simulink model "SwitchingFrequencyControlComponent"  (R2026a)
settings: Solver=FixedStepDiscrete
settings Model: DataDictionary=TractionEmotorSoftwareArchInterfaceData.sldd  Creator=dakaihu  LastModifiedBy=dakaihu

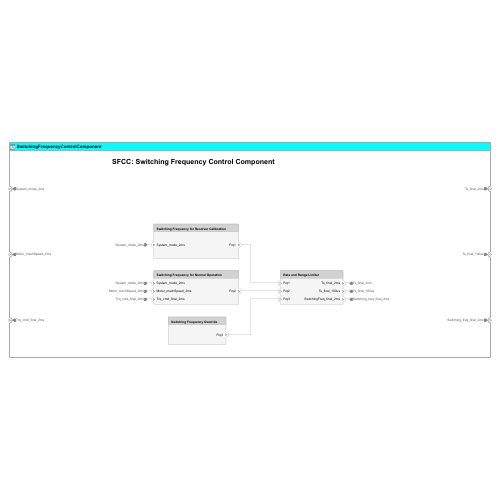
[thumbnail: Simulink's stored preview of the top-level diagram]
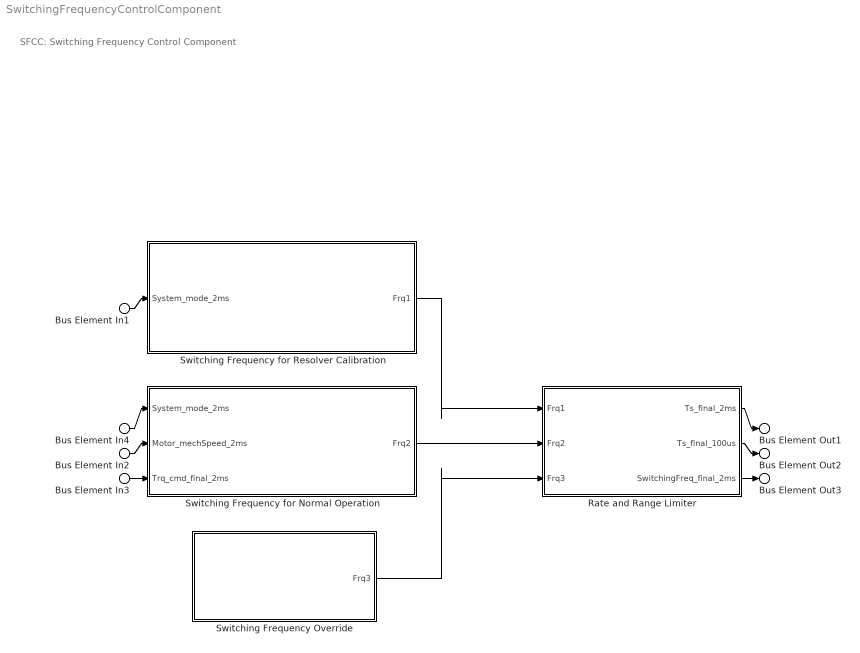
== system SwitchingFrequencyControlComponent ==
  note: SFCC: Switching Frequency Control Component
  Bus Element In1 : Inport  PortName=System_mode_2ms
  Bus Element In4 : Inport  PortName=System_mode_2ms
  Bus Element In2 : Inport  Port=2  PortName=Motor_mechSpeed_2ms
  Bus Element In3 : Inport  Port=3  PortName=Trq_cmd_final_2ms
  Rate and Range Limiter : Subsystem
      settings: PortSchema="{\"entries\":[{\"content\":{\"headerSize\":26,\"margin\":15,\"minimumSpacing\":25,\"sides\":[{\"content\":{\"connectorIds\":[\"In1\",\"In2\",\"In3\"]},\"type\":\"ConnectorPlacement.EquallySpacedRectSide\",\"uuid\":\"e09fe738-2b2d-403f-b055-60947e3a12a9\"},{\"content\":{\"connectorIds\":[\"Out1\",\"Out2\",\"Out3\"],\"side\":\"RIGHT\"},\"type\":\"ConnectorPlacement.EquallySpacedRectSide\",\"uuid\":\"7566e870-d5f8-4c16-9c2a-de0e46bcfc8a\"},{\"content\":{\"connectorIds\":[],\"side\":\"TOP\"},\"type\":\"ConnectorPlacement.EquallySpacedRectSide\",\"uuid\":\"baa3809f-6a8a-4fc9-b6be-968aafcdb1b7\"}]},\"type\":\"ConnectorPlacement.EquallySpacedConnector\",\"uuid\":\"274f79bf-3dc3-455f-a70a-3832140476bd\"}],\"packageUris\":[\"http://schema.mathworks.com/mf0/Connector/R2020b\"],\"version\":\"1.0\"}"
  Switching Frequency Override : Subsystem
      settings: PortSchema="{\"entries\":[{\"content\":{\"headerSize\":26,\"margin\":15,\"minimumSpacing\":25,\"sides\":[{\"content\":{\"connectorIds\":[]},\"type\":\"ConnectorPlacement.EquallySpacedRectSide\",\"uuid\":\"e09fe738-2b2d-403f-b055-60947e3a12a9\"},{\"content\":{\"connectorIds\":[\"Out1\"],\"side\":\"RIGHT\"},\"type\":\"ConnectorPlacement.EquallySpacedRectSide\",\"uuid\":\"7566e870-d5f8-4c16-9c2a-de0e46bcfc8a\"},{\"content\":{\"connectorIds\":[],\"side\":\"TOP\"},\"type\":\"ConnectorPlacement.EquallySpacedRectSide\",\"uuid\":\"baa3809f-6a8a-4fc9-b6be-968aafcdb1b7\"}]},\"type\":\"ConnectorPlacement.EquallySpacedConnector\",\"uuid\":\"274f79bf-3dc3-455f-a70a-3832140476bd\"}],\"packageUris\":[\"http://schema.mathworks.com/mf0/Connector/R2020b\"],\"version\":\"1.0\"}"
  Switching Frequency for Normal Operation : Subsystem
      settings: PortSchema="{\"entries\":[{\"content\":{\"headerSize\":26,\"margin\":15,\"minimumSpacing\":25,\"sides\":[{\"content\":{\"connectorIds\":[\"In1\",\"In2\",\"In3\"]},\"type\":\"ConnectorPlacement.EquallySpacedRectSide\",\"uuid\":\"e09fe738-2b2d-403f-b055-60947e3a12a9\"},{\"content\":{\"connectorIds\":[\"Out1\"],\"side\":\"RIGHT\"},\"type\":\"ConnectorPlacement.EquallySpacedRectSide\",\"uuid\":\"7566e870-d5f8-4c16-9c2a-de0e46bcfc8a\"},{\"content\":{\"connectorIds\":[],\"side\":\"TOP\"},\"type\":\"ConnectorPlacement.EquallySpacedRectSide\",\"uuid\":\"baa3809f-6a8a-4fc9-b6be-968aafcdb1b7\"}]},\"type\":\"ConnectorPlacement.EquallySpacedConnector\",\"uuid\":\"274f79bf-3dc3-455f-a70a-3832140476bd\"}],\"packageUris\":[\"http://schema.mathworks.com/mf0/Connector/R2020b\"],\"version\":\"1.0\"}"
  Switching Frequency for Resolver Calibration : Subsystem
      settings: PortSchema="{\"entries\":[{\"content\":{\"headerSize\":26,\"margin\":15,\"minimumSpacing\":25,\"sides\":[{\"content\":{\"connectorIds\":[\"In1\"]},\"type\":\"ConnectorPlacement.EquallySpacedRectSide\",\"uuid\":\"e09fe738-2b2d-403f-b055-60947e3a12a9\"},{\"content\":{\"connectorIds\":[\"Out1\"],\"side\":\"RIGHT\"},\"type\":\"ConnectorPlacement.EquallySpacedRectSide\",\"uuid\":\"7566e870-d5f8-4c16-9c2a-de0e46bcfc8a\"},{\"content\":{\"connectorIds\":[],\"side\":\"TOP\"},\"type\":\"ConnectorPlacement.EquallySpacedRectSide\",\"uuid\":\"baa3809f-6a8a-4fc9-b6be-968aafcdb1b7\"}]},\"type\":\"ConnectorPlacement.EquallySpacedConnector\",\"uuid\":\"274f79bf-3dc3-455f-a70a-3832140476bd\"}],\"packageUris\":[\"http://schema.mathworks.com/mf0/Connector/R2020b\"],\"version\":\"1.0\"}"
  Bus Element Out1 : Outport  PortName=Ts_final_2ms
  Bus Element Out2 : Outport  Port=2  PortName=Ts_final_100us
  Bus Element Out3 : Outport  Port=3  PortName=Switching_freq_final_2ms
  wires:
  Bus Element In1/1 -> Switching Frequency for Resolver Calibration/1(System_mode_2ms)
  Bus Element In2/1 -> Switching Frequency for Normal Operation/2(Motor_mechSpeed_2ms)
  Bus Element In4/1 -> Switching Frequency for Normal Operation/1(System_mode_2ms)
  Bus Element In3/1 -> Switching Frequency for Normal Operation/3(Trq_cmd_final_2ms)
  Switching Frequency for Resolver Calibration/1(Frq1) -> Rate and Range Limiter/1(Frq1)
  Switching Frequency for Normal Operation/1(Frq2) -> Rate and Range Limiter/2(Frq2)
  Switching Frequency Override/1(Frq3) -> Rate and Range Limiter/3(Frq3)
  Rate and Range Limiter/1(Ts_final_2ms) -> Bus Element Out1/1
  Rate and Range Limiter/2(Ts_final_100us) -> Bus Element Out2/1
  Rate and Range Limiter/3(SwitchingFreq_final_2ms) -> Bus Element Out3/1

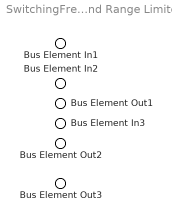
== system SwitchingFrequencyControlComponent/Rate and Range Limiter ==
  Bus Element In1 : Inport  PortName=Frq1
  Bus Element In2 : Inport  Port=2  PortName=Frq2
  Bus Element In3 : Inport  Port=3  PortName=Frq3
  Bus Element Out1 : Outport  PortName=Ts_final_2ms
  Bus Element Out2 : Outport  Port=2  PortName=Ts_final_100us
  Bus Element Out3 : Outport  Port=3  PortName=SwitchingFreq_final_2ms

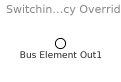
== system SwitchingFrequencyControlComponent/Switching Frequency Override ==
  Bus Element Out1 : Outport  PortName=Frq3

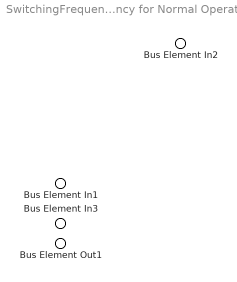
== system SwitchingFrequencyControlComponent/Switching Frequency for Normal Operation ==
  Bus Element In2 : Inport  PortName=System_mode_2ms
  Bus Element In1 : Inport  Port=2  PortName=Motor_mechSpeed_2ms
  Bus Element In3 : Inport  Port=3  PortName=Trq_cmd_final_2ms
  Bus Element Out1 : Outport  PortName=Frq2

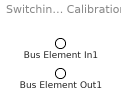
== system SwitchingFrequencyControlComponent/Switching Frequency for Resolver Calibration ==
  Bus Element In1 : Inport  PortName=System_mode_2ms
  Bus Element Out1 : Outport  PortName=Frq1
